simulink model "p_inv_sub_coupled_CI_1"  (Simulink 9.0)
settings: Solver=ode45  StartTime=0.0  StopTime=300  FixedStep=0.0001  MaxStep=0.001  RelTol=1e-6  AbsTol=1e-6
values from neighbouring files (symbols this model uses):
  CI1_sim = CI1(jj)    [erick_main_CI_1.m]
  CI2_sim = CI2(ii)    [erick_main_CI_1.m]
settings Model: Creator=Erick  LastModifiedBy=Erick
settings DataIOCC: SaveFormat=Dataset
settings OptimizationCC: LifeSpan=auto
settings DebuggingCC: UnderspecifiedInitializationDetection=Simplified  MergeDetectMultiDrivingBlocksExec=error  SFUnexpectedBacktrackingDiag=error  SFNoUnconditionalDefaultTransitionDiag=error  SFExecutionAtInitializationDiag=warning
settings HardwareCC: ProdBitPerPointer=64  ProdBitPerSizeT=64  ProdBitPerPtrDiffT=64  ProdLargestAtomicFloat=Float  ProdIntDivRoundTo=Zero  ProdEndianess=LittleEndian  ProdWordSize=64  ProdHWDeviceType=Intel->x86-64 (Windows64)
settings ModelReferenceCC: PropagateSignalLabelsOutOfModel=on
settings CodeAppCC: StateflowObjectComments=off
settings GRTTargetCC: TargetLangStandard=C99 (ISO)
settings ConfigComp: CovMetricSettings=dwe  CovHtmlReporting=off  CovSaveCumulativeToWorkspaceVar=off  CovSaveSingleToWorkspaceVar=off  CovExternalEMLEnable=on

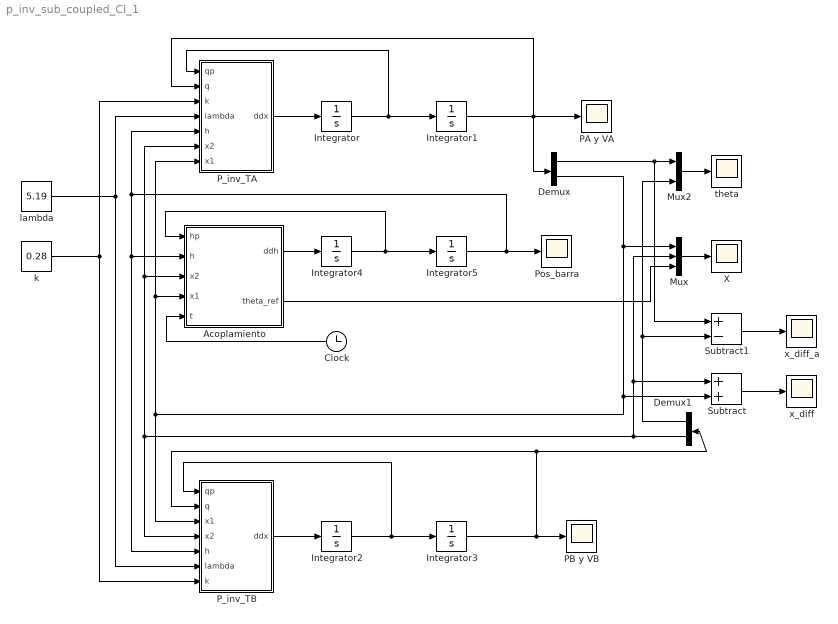
== system p_inv_sub_coupled_CI_1 ==
  Acoplamiento : MATLAB Function  TreatAsAtomicUnit=on
  Clock : Clock
  Demux : Demux  Outputs=2
  Demux1 : Demux  Outputs=2
  Integrator : Integrator  InitialCondition=[0 0]
  Integrator1 : Integrator  InitialCondition="[CI1_sim  0]"
  Integrator2 : Integrator  InitialCondition=[0 0]
  Integrator3 : Integrator  InitialCondition="[CI2_sim  0]"
  Integrator4 : Integrator
  Integrator5 : Integrator
  Mux : Mux  Inputs=3
  Mux2 : Mux  Inputs=2
  PA y VA : Scope
  PB y VB : Scope
  P_inv_TA : MATLAB Function  TreatAsAtomicUnit=on
  P_inv_TB : MATLAB Function  TreatAsAtomicUnit=on
  Pos_barra : Scope
  Subtract : Sum
  Subtract1 : Sum  Inputs=+-
  X : Scope
  k : Constant  Value=0.28
  lambda : Constant  Value=5.19
  theta : Scope
  x_diff : Scope
  x_diff_a : Scope
  wires:
  P_inv_TA/1(ddx) -> Integrator/1
  Integrator1/1 -> P_inv_TA/2(q), PA y VA/1, Demux/1
  Integrator/1 -> Integrator1/1, P_inv_TA/1(qp)
  Integrator2/1 -> P_inv_TB/1(qp), Integrator3/1
  P_inv_TB/1(ddx) -> Integrator2/1
  Integrator3/1 -> Demux1/1, P_inv_TB/2(q), PB y VB/1
  Integrator4/1 -> Acoplamiento/1(hp), Integrator5/1
  Acoplamiento/1(ddh) -> Integrator4/1
  Integrator5/1 -> Pos_barra/1, P_inv_TB/5(h), Acoplamiento/2(h), P_inv_TA/5(h)
  Mux/1 -> X/1
  Demux/2 -> Subtract/2, Acoplamiento/4(x1), P_inv_TA/7(x1), P_inv_TB/3(x1), Mux/1
  Demux1/2 -> Mux/2, Subtract/1, Acoplamiento/3(x2), P_inv_TA/6(x2), P_inv_TB/4(x2)
  Clock/1 -> Acoplamiento/5(t)
  Acoplamiento/2(theta_ref) -> Mux/3
  Mux2/1 -> theta/1
  Demux/1 -> Subtract1/1, Mux2/1
  lambda/1 -> P_inv_TB/6(lambda), P_inv_TA/4(lambda)
  Subtract/1 -> x_diff/1
  Subtract1/1 -> x_diff_a/1
  Demux1/1 -> Mux2/2, Subtract1/2
  k/1 -> P_inv_TB/7(k), P_inv_TA/3(k)

== matlab function P_inv_TB ==
  data: qp input double; q input double; x1 input double; x2 input double; ddx output double; h input double; lambda input double; k input double
function ddx = fcn(qp,q,x1,x2,h,lambda,k)
% function ddx = fcn(qp,q,h,x1,x2)

theta = q(1);
x = q(2);
thetap = qp(1);
xp = qp(2);

% parametros
g = 9.81;       % m/s^2
m1 = 1.785;     % kg
m2 = 0.213;     % kg
l1 = 0.330;     % m
lc1 = -0.0376;  % m
I1I2 = 0.0246;  % kgm^2

% parámetros para resultados numericos
k1 = 2.2409;
k2 = 2.1235;
k3 = 0.1854;
k4 = 1.5353;

% lambda =  5.5;   
gamma = 0.2025;
% gamma = 0.1163;
% sigma = 5;
% sigma = 20; % sincro mas rapido pero no sincro en antifase
sigma = 0;
% k = 0.251;

% Señal de control
u = -k1*theta-k2*x-k3*thetap-k4*xp-lambda*(x^2+xp^2-gamma)*xp+k*(x2+x1)+sigma*h;
% u = 0;

M = [I1I2+(x^2+l1^2)*m2-m1*lc1^2 l1*m2;
     l1*m2 m2]; % Matriz de inercia

C = [2*m2*x*xp 0;
    -m2*thetap*x 0]*[thetap;xp]; % Matriz de coriolis

G=[-m2*g*cos(theta)*x-(l1*m2+m1*lc1)*g*sin(theta);
    -m2*g*sin(theta)]; % Matriz de fuerzas gravitacionales

tau = [0; u]; % torque de control (sub actuado)
F = tau-C-G; 

ddx = inv(M)*F;

== matlab function P_inv_TA ==
  data: qp input double; q input double; k input double; lambda input double; h input double; x2 input double; x1 input double; ddx output double
function ddx = fcn(qp,q,k,lambda,h,x2,x1)
% function ddx = fcn(qp,q,x1,x2,h)

theta = q(1);
x = q(2);
thetap = qp(1);
xp = qp(2);

% parametros
g = 9.81;       % m/s^2
m1 = 1.785;     % kg
m2 = 0.213;     % kg
l1 = 0.330;     % m
lc1 = -0.0376;  % m
I1I2 = 0.0246;  % kgm^2

% parámetros para resultados numericos
k1 = 2.2409;
k2 = 2.1235;
k3 = 0.1854;
k4 = 1.5353;

% lambda =  5.5;  % ?   
gamma = 0.2025;
% gamma = 0.1163;
% sigma = 5;
% sigma = 20; % sincro mas rapido pero no sincro en antifase
sigma = 0;
% k = 0.251;


% Señal de control
u = -k1*theta-k2*x-k3*thetap-k4*xp-lambda*(x^2+xp^2-gamma)*xp+k*(x1+x2)+sigma*h;

M = [I1I2+(x^2+l1^2)*m2-m1*lc1^2 l1*m2;
     l1*m2 m2]; % Matriz de inercia

C = [2*m2*x*xp 0;
    -m2*thetap*x 0]*[thetap;xp]; % Matriz de coriolis

G=[-m2*g*cos(theta)*x-(l1*m2+m1*lc1)*g*sin(theta);
    -m2*g*sin(theta)]; % Matriz de fuerzas gravitacionales

tau = [0;u]; % torque de control (sub actuado)
   
% Fric_viscosa = 0.01*qp; % no esta en el modelo, es para probar

F = tau-C-G; 
% F = tau+C*[thetap;xp]+G+Fric_viscosa; 

ddx = inv(M)*F;

== matlab function Acoplamiento ==
  data: hp input double; h input double; x2 input double; ddh output double; x1 input double; t input double; theta_ref output double
function [ddh,theta_ref] = fcn(hp,h,x2,x1,t)

% parametros
h1=45;  % r1
h2=3.1; % r2
% h1 = 0.4094;
% h2 = 0.4094;
mu=.35; % ?


% eta = 0.06; % ?
% w = 5.4611; % ?
% w = 6.2;


g = 9.81;       % m/s^2
m1 = 1.785;     % kg
m2 = 0.213;     % kg
l1 = 0.330;     % m
lc1 = -0.0376;  % m
I1I2 = 0.0246;  % kgm^2


% w = 6.6887;
% w = 6.0357;
% w = 6.0415;
w = 6.0357;
% eta = 0.0164142;
eta = 0.024496;
% eta = 0.034456;
theta_ref = eta*sin(w*t);


% theta_refp = eta*w*cos(w*t);
% theta_refpp = -eta*w^2*sin(w*t);

% F = 2*m1*lc1*(theta_refpp*cos(theta_ref)-theta_refp^2*sin(theta_ref));

ddh=-h1*h-h2*hp+mu*(x1+x2-2*theta_ref);
